simulink model "CLIK_con_inversa"  (R2022b)
settings: Solver=VariableStepAuto  StartTime=0.0  StopTime=40  RelTol=1e-3
values from neighbouring files (symbols this model uses):
  k_inversa = 10    [CLIK_script.m]
  T = T_A * T_B    [DH_dinamica.m]    (also in traiettoria_script.m = 0.001)
  theta1_0 = pi/2 - angolo    [CLIK_script.m]
  theta2_0 = 2*angolo    [CLIK_script.m]
undefined symbols (not defined in the file or in its folder): DiscIntNeverNeededParam
libraries: simulink x1
settings Model: Creator=Michele  LastModifiedBy=Michele
settings DataIOCC: ReturnWorkspaceOutputs=off

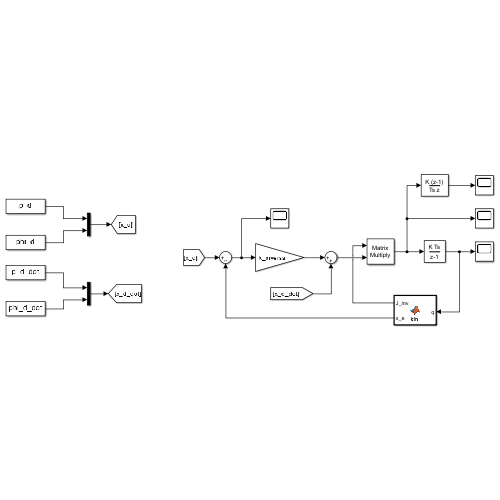
[thumbnail: Simulink's stored preview of the top-level diagram]
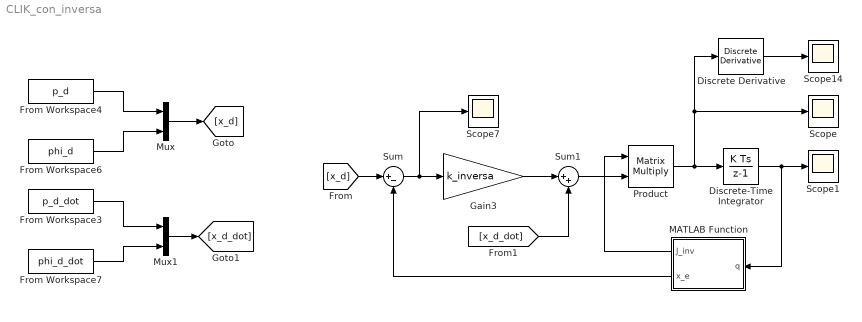
== system CLIK_con_inversa ==
  Discrete Derivative : simulink/Discrete/Discrete Derivative  gainval=1.0  ICPrevScaledInput=[0 0 0 0]'  OutMin=[]  OutMax=[]  OutDataType=fixdt(1, 16)  OutScaling=2^-10  DoSatur=off
  Discrete-Time Integrator : DiscreteIntegrator  InitialCondition=[theta1_0 theta2_0 -0.25 0]'  SampleTime=-1  ICPrevOutput=DiscIntNeverNeededParam  ICPrevScaledInput=DiscIntNeverNeededParam
  From Workspace3 : FromWorkspace  VariableName=p_d_dot  SampleTime=T
  From Workspace4 : FromWorkspace  VariableName=p_d  SampleTime=T
  From Workspace6 : FromWorkspace  VariableName=phi_d  SampleTime=T
  From Workspace7 : FromWorkspace  VariableName=phi_d_dot  SampleTime=T
  Gain3 : Gain  Gain=k_inversa
  MATLAB Function : MATLAB Function  TreatAsAtomicUnit=on
  Mux : Mux  Inputs=2
  Mux1 : Mux  Inputs=2
  Product : Product  Multiplication=Matrix(*)
  Scope{,1,7,14} (4 alike) : Scope
  Sum : Sum  Inputs=|+-
  Sum1 : Sum  Inputs=|++
  wires:
  MATLAB Function/2(x_e) -> Sum/2
  Sum/1 -> Scope7/1, Gain3/1
  [x_d_dot] -> Sum1/2
  Gain3/1 -> Sum1/1
  Sum1/1 -> Product/2
  MATLAB Function/1(J_inv) -> Product/1
  Discrete Derivative/1 -> Scope14/1
  [x_d] -> Sum/1
  Product/1 -> Discrete-Time Integrator/1, Discrete Derivative/1, Scope/1
  Discrete-Time Integrator/1 -> Scope1/1, MATLAB Function/1(q)
  Mux1/1 -> [x_d_dot]
  From Workspace3/1 -> Mux1/1
  Mux/1 -> [x_d]
  From Workspace7/1 -> Mux1/2
  From Workspace4/1 -> Mux/1
  From Workspace6/1 -> Mux/2

== matlab function CLIK_con_inversa/MATLAB Function ==
  data: J_inv output; q input; x_e output
function [J_inv,x_e] = kin(q)
    
    q1 = q(1); q2 = q(2); q3 = q(3); q4 = q(4);

    J = [- sin(q1)/2 - (cos(q1)*sin(q2))/2 - (cos(q2)*sin(q1))/2, - (cos(q1)*sin(q2))/2 - (cos(q2)*sin(q1))/2, 0, 0;
           cos(q1)/2 + (cos(q1)*cos(q2))/2 - (sin(q1)*sin(q2))/2,   (cos(q1)*cos(q2))/2 - (sin(q1)*sin(q2))/2, 0, 0;
                                                               0,                                           0, 1, 0;
                                                               0,                                           0, 0, 1];

    x_e = [cos(q1)/2 + (cos(q1)*cos(q2))/2 - (sin(q1)*sin(q2))/2;
           sin(q1)/2 + (cos(q1)*sin(q2))/2 + (cos(q2)*sin(q1))/2;
                                                   q3;
                                                   q4];
    
    J_inv= inv(J);
end
